simulink model "Pract4Simu"  (R2025a)
settings: Solver=VariableStepAuto  StartTime=0.0  StopTime=10.0  MaxStep=0.01  RelTol=1e-3
InitFcn:
  | m = 10;
  | k = 100;
  | r = 0.05;

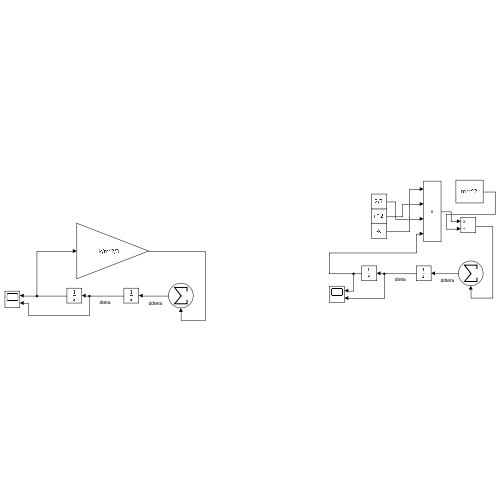
[thumbnail: Simulink's stored preview of the top-level diagram]
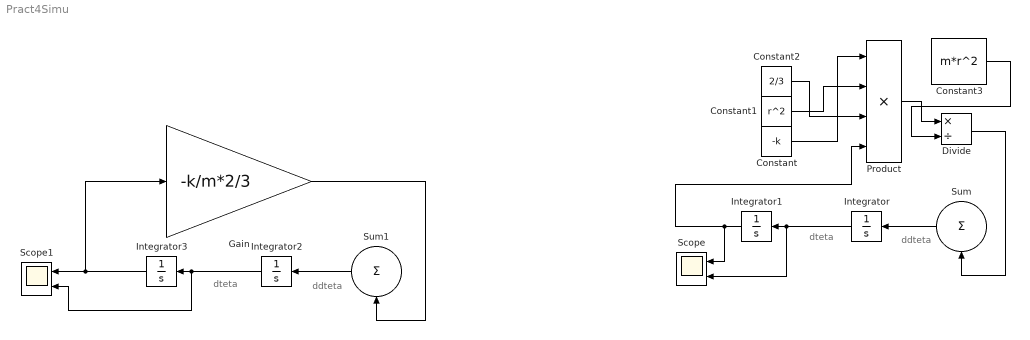
== system Pract4Simu ==
  note: dteta
  note: ddteta
  note: dteta
  note: ddteta
  Constant : Constant  Value=-k
  Constant1 : Constant  Value=r^2
  Constant2 : Constant  Value=2/3
  Constant3 : Constant  Value=m*r^2
  Divide : Product  Inputs=*/
  Gain : Gain  Gain=-k/m*2/3
  Integrator : Integrator  InitialCondition=2
  Integrator1 : Integrator
  Integrator2 : Integrator  InitialCondition=2
  Integrator3 : Integrator
  Product : Product  Inputs=4
  Scope : Scope  NumInputPorts=2
      settings: ActiveDisplayYMinimum=-2.4999977040404779  ActiveDisplayYMaximum=2.4999997448933864
  Scope1 : Scope  NumInputPorts=2
      settings: ActiveDisplayYMinimum=-2.4999977040404797  ActiveDisplayYMaximum=2.4999997448933864
  Sum : Sum  Inputs=|+
  Sum1 : Sum  Inputs=|+
  wires:
  Integrator/1 -> Scope/2, Integrator1/1
  Sum/1 -> Integrator/1
  Integrator1/1 -> Product/4, Scope/1
  Constant/1 -> Product/1
  Constant1/1 -> Product/2
  Constant2/1 -> Product/3
  Product/1 -> Divide/1
  Constant3/1 -> Divide/2
  Divide/1 -> Sum/1
  Integrator2/1 -> Scope1/2, Integrator3/1
  Integrator3/1 -> Gain/1, Scope1/1
  Gain/1 -> Sum1/1
  Sum1/1 -> Integrator2/1
